simulink model "rf_bb_1"  (Simulink 7.4)
settings: Solver=ode45  SolverMode=SingleTasking  StartTime=0.0  StopTime=200e-5  RelTol=1e-6
undefined symbols (not defined in the file or in its folder): Fs, magnitude
libraries: dspindex x6, dsparch4 x4, dspsigops x3, dspbuff3 x2, dspxfrm3 x2, dsparch3 x2, dspsnks4 x2, dspmtrx3 x1, simulink x1
settings Model: Creator=Owner  LastModifiedBy=Dick
settings DataIOCC: SaveOutput=off  SaveTime=off
settings OptimizationCC: BooleanDataType=off  InlineInvariantSignals=on  InitFltsAndDblsToZero=on
settings DebuggingCC: SaveWithParameterizedLinksMsg=none  SignalResolutionControl=TryResolveAllWithWarning  SolverPrmCheckMsg=none  MultiTaskDSMMsg=warning  MultiTaskCondExecSysMsg=none  StrictBusMsg=None
settings HardwareCC: TargetUnknown=on
settings RTWCC: IncludeERTFirstTime=on
settings GRTTargetCC: TargetFcnLib=ansi_tfl_tmw.mat

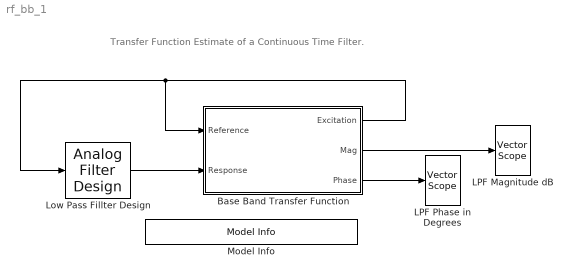
== system rf_bb_1 ==
  note: Transfer Function Estimate of a Continuous Time Filter.
  Base Band Transfer Function : Subsystem  Description=Spectrum Analyzer  mask{BW=5e6, NFFT=1024, Avg_fac=100}
      mask prompts: BW "Bandwidth"; NFFT "FFT Length (power of 2)"; Avg_fac "Averaging Factor (>=1)"
  LPF Magnitude dB : dspsnks4/Vector Scope  DialogController=dspdialog.VectorScope  DialogControllerArgs=DataTag5  ScopeProperties=on  Domain=Frequency  HorizSpan=1  DisplayProperties=off  AxisGrid=on  Memory=off  FrameNumber=on  AxisLegend=off  AxisZoom=off  OpenScopeAtSimStart=on  OpenScopeImmediately=off  FigPos=[15 321 372 236]  AxisProperties=off  XUnits=Hertz  XRange=[0...Fs/2]  InheritXIncr=on  XIncr=2*Fs  XLabel=Time  XLimit=Auto  XMin=0  XMax=1  XStart=0  YUnits=dB  YLabel=dB  LineProperties=off  LineColors=[1 0 0]|[1 0 0]  XAxisParamsVer=6.8
      settings: YMin=-100  YMax=10
  LPF Phase in Degrees : dspsnks4/Vector Scope  DialogController=dspdialog.VectorScope  DialogControllerArgs=DataTag6  ScopeProperties=on  Domain=Frequency  HorizSpan=1  DisplayProperties=off  AxisGrid=on  Memory=off  FrameNumber=on  AxisLegend=off  AxisZoom=off  OpenScopeAtSimStart=on  OpenScopeImmediately=off  FigPos=[16 37 372 236]  AxisProperties=off  XUnits=Hertz  XRange=[0...Fs/2]  InheritXIncr=on  XIncr=1  XLabel=Frequency  XLimit=Auto  XMin=0  XMax=1  XStart=0  YUnits=Magnitude  YLabel=Phase in Degrees  LineProperties=off  LineColors=[1 0 0]  XAxisParamsVer=6.8
      settings: YMin=-1000  YMax=0
  Low Pass Fillter Design : dsparch4/Analog Filter Design  method=Elliptic  filttype=Lowpass  N=8  Wlo=1e6*2*pi  Whi=80  Rp=1  Rs=90
  Model Info : simulink/Model-Wide Utilities/Model Info  SystemSampleTime=-1  InitialBlockCM=None  BlockCM=None  Frame=on  DisplayStringWithTags=Copywrite 2005-2010 The MathWorks, Inc.  HorizontalTextAlignment=Center  LeftAlignmentValue=0.5  SourceBlockDiagram=rf_bb_1  TagMaxNumber=20
  wires:
  Low Pass Fillter Design/1 -> Base Band Transfer Function/2(Response)
  Base Band Transfer Function/1(Excitation) -> Low Pass Fillter Design/1, Base Band Transfer Function/1("Reference ")
  Base Band Transfer Function/2(Mag) -> LPF Magnitude dB/1
  Base Band Transfer Function/3(Phase) -> LPF Phase in Degrees/1

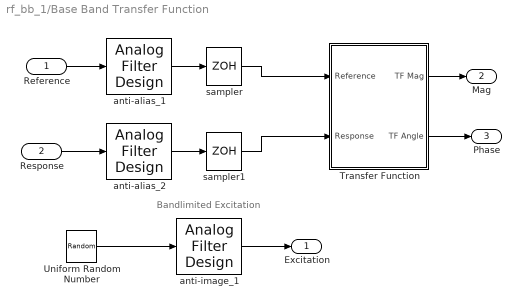
== system rf_bb_1/Base Band Transfer Function ==
  note: Bandlimited Excitation
  "Reference " : Inport  OutDataType=sfix(16)  OutScaling=2^0
  Response : Inport  Port=2  OutDataType=sfix(16)  OutScaling=2^0
  "Transfer Function " : Subsystem  mask{NFFT=NFFT, Navg=Avg_fac, pcnt=100/1.28, unwrap_flag=on}
      mask prompts: NFFT "FFT length (power of 2):"; Navg "Spectral Averaging Factor (>=1):"; pcnt "Percentage of  Alias Free Data  (<=100)"; unwrap_flag "Unwrap Phase"
      mask Display: disp('Transfer Function \n Estimation (v2.0) ')
  Uniform Random Number : UniformRandomNumber  SampleTime=1/(2.56*BW)
  anti-alias_1 : dsparch4/Analog Filter Design  method=Elliptic  filttype=Lowpass  N=8  Wlo=BW*2*pi  Whi=80  Rp=2  Rs=100
  anti-alias_2 : dsparch4/Analog Filter Design  method=Elliptic  filttype=Lowpass  N=8  Wlo=BW*2*pi  Whi=80  Rp=2  Rs=100
  anti-image_1 : dsparch4/Analog Filter Design  method=Elliptic  filttype=Lowpass  N=8  Wlo=BW*2*pi  Whi=80  Rp=2  Rs=100
  sampler : ZeroOrderHold  SampleTime=1/(2.56*BW)
  sampler1 : ZeroOrderHold  SampleTime=1/(2.56*BW)
  Excitation : Outport  OutDataType=sfix(16)  OutScaling=2^0
  Mag : Outport  Port=2  OutDataType=sfix(16)  OutScaling=2^0
  Phase : Outport  Port=3  OutDataType=sfix(16)  OutScaling=2^0
  wires:
  "Transfer Function "/2(TF Angle) -> Phase/1
  "Transfer Function "/1(TF Mag) -> Mag/1
  sampler1/1 -> "Transfer Function "/2(Response)
  sampler/1 -> "Transfer Function "/1(Reference)
  anti-image_1/1 -> Excitation/1
  Uniform Random Number/1 -> anti-image_1/1
  Response/1 -> anti-alias_2/1
  anti-alias_2/1 -> sampler1/1
  "Reference "/1 -> anti-alias_1/1
  anti-alias_1/1 -> sampler/1

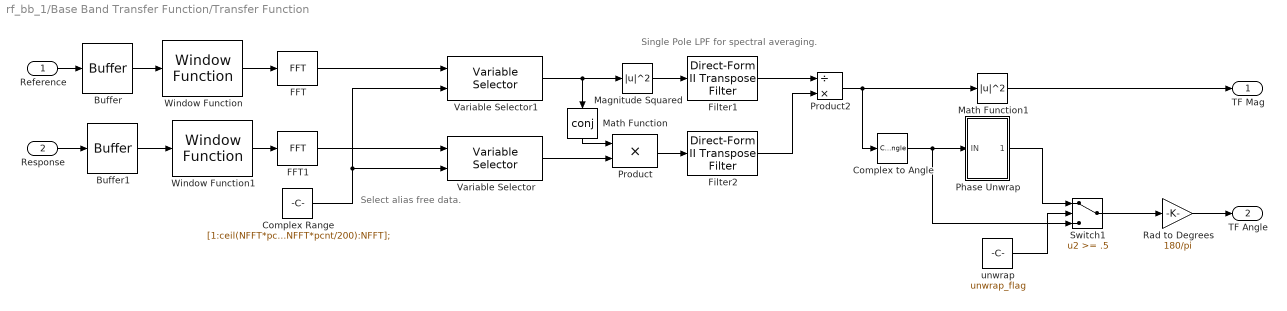
== system rf_bb_1/Base Band Transfer Function/Transfer Function  ==
  note: Single Pole LPF for spectral averaging.
  note: Select alias free data.
  Reference : Inport  OutDataType=sfix(16)  OutScaling=2^0
  Response : Inport  Port=2  OutDataType=sfix(16)  OutScaling=2^0
  Buffer : dspbuff3/Buffer  N=NFFT  V=0  ic=0
  Buffer1 : dspbuff3/Buffer  N=NFFT  V=0  ic=0
  Complex Range : Constant  Value=[1:ceil(NFFT*pcnt/200),ceil(1+NFFT-NFFT*pcnt/200):NFFT];  OutDataType=sfix(16)  OutScaling=2^0
  Complex to Angle : ComplexToMagnitudeAngle  Output=Angle
  FFT : dspxfrm3/FFT  DialogController=dspDDGCreate  DialogControllerArgs=DataTag0  CompMethod=Table lookup  TableOpt=HYBRID  TableOptActive=Speed  BitRevOrder=off  InheritFFTLength=on  FFTLength=64  SkipNorm=on  firstCoeffMode=Specify word length  firstCoeffWordLength=16  firstCoeffFracLength=15  roundingMode=Floor  overflowMode=off
  FFT1 : dspxfrm3/FFT  DialogController=dspDDGCreate  DialogControllerArgs=DataTag1  CompMethod=Table lookup  TableOpt=HYBRID  TableOptActive=Speed  BitRevOrder=off  InheritFFTLength=on  FFTLength=64  SkipNorm=on  firstCoeffMode=User-defined  firstCoeffWordLength=16  firstCoeffFracLength=15  roundingMode=Floor  overflowMode=off
  Filter1 : dsparch3/Direct-Form II Transpose Filter  num=1  den=[Navg -(Navg-1)]  ic=eps
  Filter2 : dsparch3/Direct-Form II Transpose Filter  num=1  den=[Navg -(Navg-1)]  ic=eps
  Magnitude Squared : Math  Operator=magnitude^2  OutDataType=sfix(16)  OutScaling=2^0  SaturateOnIntegerOverflow=on
  Math Function : Math  Operator=conj  OutDataType=sfix(16)  OutScaling=2^0  SaturateOnIntegerOverflow=on
  Math Function1 : Math  Operator=magnitude^2  OutDataType=sfix(16)  OutScaling=2^0  SaturateOnIntegerOverflow=on
  Phase Unwrap : Subsystem
  Product : Product  OutDataType=sfix(16)  OutScaling=2^0  SaturateOnIntegerOverflow=on  InputSameDT=on  OutDataTypeStr=Inherit: Same as first input
  Product2 : Product  Inputs=/*  OutDataType=sfix(16)  OutScaling=2^0  SaturateOnIntegerOverflow=on  InputSameDT=on  OutDataTypeStr=Inherit: Same as first input
  Rad to Degrees : Gain  Gain=180/pi  ParameterDataType=sfix(16)  ParameterScaling=2^0  OutDataType=sfix(16)  OutScaling=2^0
  Switch1 : Switch  Threshold=.5
  Variable Selector : dspindex/Variable Selector  NumInputs=1  rowsOrCols=Rows  IdxMode=Variable  Elements=[1 3]  ZerOneIdxMode=One-based  errmode=Clip Index  FillMode=on  FillValues=0
  Variable Selector1 : dspindex/Variable Selector  NumInputs=1  rowsOrCols=Rows  IdxMode=Variable  Elements=[1 3]  ZerOneIdxMode=One-based  errmode=Clip Index  FillMode=on  FillValues=0
  Window Function : dspsigops/Window Function  DialogController=dspDDGCreate  DialogControllerArgs=DataTag3  winmode=Apply window to input  wintype=Hann  sampmode=Continuous  samptime=1  N=64  Rs=50  beta=10  winsamp=Periodic  UserWindow=hamming  OptParams=off  UserParams={'symmetric'}  dataType=double  isSigned=on  wordLen=16  udDataType=sfix(16)  fracBitsMode=Best precision  numFracBits=15  roundingMode=Floor  overflowMode=off  numSidelobes=4  sidelobeLevel=-30
  Window Function1 : dspsigops/Window Function  DialogController=dspDDGCreate  DialogControllerArgs=DataTag4  winmode=Apply window to input  wintype=Hann  sampmode=Continuous  samptime=1  N=64  Rs=50  beta=10  winsamp=Periodic  UserWindow=hamming  OptParams=off  UserParams={'symmetric'}  dataType=double  isSigned=on  wordLen=16  udDataType=sfix(16)  fracBitsMode=Best precision  numFracBits=15  roundingMode=Floor  overflowMode=off  numSidelobes=4  sidelobeLevel=-30
  unwrap : Constant  Value=unwrap_flag  OutDataType=sfix(16)  OutScaling=2^0
  TF Mag : Outport  OutDataType=sfix(16)  OutScaling=2^0
  TF Angle : Outport  Port=2  OutDataType=sfix(16)  OutScaling=2^0
  wires:
  Complex Range/1 -> Variable Selector/2, Variable Selector1/2
  Complex to Angle/1 -> Switch1/3, Phase Unwrap/1(IN)
  Rad to Degrees/1 -> TF Angle/1
  Response/1 -> Buffer1/1
  Reference/1 -> Buffer/1
  Product/1 -> Filter2/1
  FFT1/1 -> Variable Selector/1
  Math Function/1 -> Product/1
  Magnitude Squared/1 -> Filter1/1
  FFT/1 -> Variable Selector1/1
  Math Function1/1 -> TF Mag/1
  Window Function/1 -> FFT/1
  Window Function1/1 -> FFT1/1
  Filter1/1 -> Product2/1
  Filter2/1 -> Product2/2
  Buffer/1 -> Window Function/1
  Buffer1/1 -> Window Function1/1
  Product2/1 -> Complex to Angle/1, Math Function1/1
  Variable Selector/1 -> Product/2
  Variable Selector1/1 -> Magnitude Squared/1, Math Function/1
  Switch1/1 -> Rad to Degrees/1
  unwrap/1 -> Switch1/2
  Phase Unwrap/1(Out1) -> Switch1/1

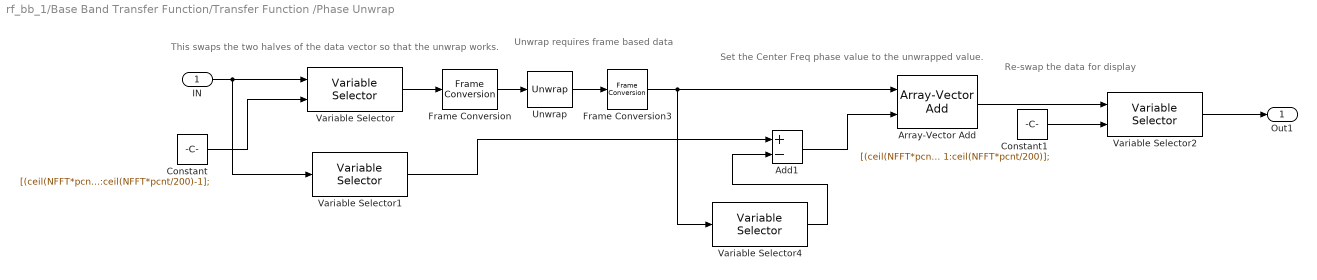
== system rf_bb_1/Base Band Transfer Function/Transfer Function /Phase Unwrap ==
  note: This swaps the two halves of the data vector
      | so that the unwrap works.
  note: Set the Center Freq phase value to the unwrapped value.
  note: Re-swap the data for display
  note: Unwrap requires frame based data
  IN : Inport  OutDataType=sfix(16)  OutScaling=2^0
  Add1 : Sum  Inputs=+-  OutDataType=sfix(16)  OutScaling=2^-10
  Array-Vector Add : dspmtrx3/Array-Vector Add  DialogController=dspDDGCreate  DialogControllerArgs=DataTag2  Dimension=2  V_Source=Input port  V_VectFromMask=[0.5 0.25]  firstCoeffDataTypeStr=Inherit: Same word length as input  firstCoeffLastDataTypeStr=Inherit: Same word length as input  firstCoeffMin=[]  firstCoeffMax=[]  outputDataTypeStr=Inherit: Same as accumulator  outputLastDataTypeStr=Inherit: Same as accumulator  outputMin=[]  outputMax=[]  roundingMode=Floor  overflowMode=off
  Constant : Constant  Value=[(ceil(NFFT*pcnt/200)):ceil(NFFT*pcnt/100) 1:ceil(NFFT*pcnt/200)-1];  OutDataType=sfix(16)  OutScaling=2^0
  Constant1 : Constant  Value=[(ceil(NFFT*pcnt/200)+1):ceil(NFFT*pcnt/100) 1:ceil(NFFT*pcnt/200)];  OutDataType=sfix(16)  OutScaling=2^0
  Frame Conversion : FrameConversion
  Frame Conversion3 : FrameConversion  OutFrame=Sample-based
  Unwrap : dspsigops/Unwrap  running=on  tol=pi
  Variable Selector : dspindex/Variable Selector  NumInputs=1  rowsOrCols=Rows  IdxMode=Variable  Elements=[1 3]  ZerOneIdxMode=One-based  errmode=Clip Index  FillMode=on  FillValues=0
  Variable Selector1 : dspindex/Variable Selector  NumInputs=1  rowsOrCols=Rows  IdxMode=Fixed  Elements=[1]  ZerOneIdxMode=One-based  errmode=Clip Index  FillMode=on  FillValues=0
  Variable Selector2 : dspindex/Variable Selector  NumInputs=1  rowsOrCols=Rows  IdxMode=Variable  Elements=[1 3]  ZerOneIdxMode=One-based  errmode=Clip Index  FillMode=on  FillValues=0
  Variable Selector4 : dspindex/Variable Selector  NumInputs=1  rowsOrCols=Rows  IdxMode=Fixed  Elements=length([(ceil(NFFT*pcnt/200)+1):ceil(NFFT*pcnt/100) 1:ceil(NFFT*pcnt/200)] )/2+1  ZerOneIdxMode=One-based  errmode=Clip Index  FillMode=on  FillValues=0
  Out1 : Outport  OutDataType=sfix(16)  OutScaling=2^0
  wires:
  Frame Conversion/1 -> Unwrap/1
  Variable Selector2/1 -> Out1/1
  IN/1 -> Variable Selector/1, Variable Selector1/1
  Constant/1 -> Variable Selector/2
  Variable Selector/1 -> Frame Conversion/1
  Variable Selector1/1 -> Add1/1
  Unwrap/1 -> Frame Conversion3/1
  Variable Selector4/1 -> Add1/2
  Constant1/1 -> Variable Selector2/2
  Frame Conversion3/1 -> Variable Selector4/1, Array-Vector Add/1
  Add1/1 -> Array-Vector Add/2
  Array-Vector Add/1 -> Variable Selector2/1
